simulink model "velo_pi_mbd_sl"  (R2023b)
settings: Solver=ode4  StartTime=0.0  StopTime=10  FixedStep=ts  RelTol=1e-3  EnableMultiTasking=on
values from neighbouring files (symbols this model uses):
  K = 0.625269    [model_data.mat]    (also in velo_id_verify.m)
  Ki = p1*p2*T/K    [velo_pi_mbd.m]
  Kp = - (T*(p1+p2)+1)/K    [velo_pi_mbd.m]
  T = 0.26    [model_data.mat]    (also in velo_id_verify.m)
  ts = 1/50    (= 0.02)    [velo_id_gain.m]    (also in velo_id_gain_cp.m; velo_id_tc.m; velo_pi_mbd.m)
  u_offset = 1.15936    [model_data.mat]    (also in velo_id_gain.m = -P(2) / P(1); velo_id_tc.m = (K_id*r_const - c1)/K_id; velo_id_verify.m)
libraries: arduinolib x2
settings Model: ExtModeTrigDuration=2  Creator=morita  LastModifiedBy=MunoLike
settings SolverCC: AlgebraicLoopSolver=TrustRegion
settings DataIOCC: SaveFormat=Array  ReturnWorkspaceOutputs=off
settings OptimizationCC: LifeSpan=1  MaxStackSize=64
settings DebuggingCC: UnconnectedInputMsg=warning  UnconnectedOutputMsg=warning  UnconnectedLineMsg=warning  SFUnexpectedBacktrackingDiag=warning  SFNoUnconditionalDefaultTransitionDiag=warning  ArithmeticOperatorsInVariantConditions=warning
settings HardwareCC: ProdBitPerInt=16  ProdBitPerPointer=16  ProdBitPerSizeT=16  ProdBitPerPtrDiffT=16  ProdLargestAtomicFloat=None  ProdWordSize=8  ProdHWDeviceType=Atmel->AVR  UseEmbeddedCoderFeatures=off  UseSimulinkCoderFeatures=off
settings ModelReferenceCC: EnableRefExpFcnMdlSchedulingChecks=on
settings SFSimCC: SimUseLocalCustomCode=off  CustomCodeUndefinedFunction=UseInterfaceOnly
settings RTWCC: Description=Embedded Coder  SystemTargetFile=ert.tlc  HardwareBoard=Arduino Uno  TemplateMakefile=ert_default_tmf  GenerateReport=on  RTWUseLocalCustomCode=off  Toolchain=Arduino AVR  BuildConfiguration=Faster Runs  LaunchReport=on
settings CodeAppCC: ForceParamTrailComments=on  OperatorAnnotations=on  StateflowObjectComments=on  MATLABSourceComments=on
settings ERTTargetCC: MultiwordLength=2048  ERTCustomFileBanners=off  SupportContinuousTime=on  SupportNonInlinedSFcns=on  SupportVariableSizeSignals=on  ModelStepFunctionPrototypeControlCompliant=off  ExtModeTransport=3  ExtModeStaticAlloc=on  ExtModeAutomaticAllocSize=off  ExtModeStaticAllocSize=250  ExtModeMexFile=ext_xcp  ExtModeIntrfLevel=Level2 - Open
settings ConfigComp: CovMetricSettings=dw  CovSaveCumulativeToWorkspaceVar=on  CovSaveSingleToWorkspaceVar=on  CovExternalEMLEnable=off

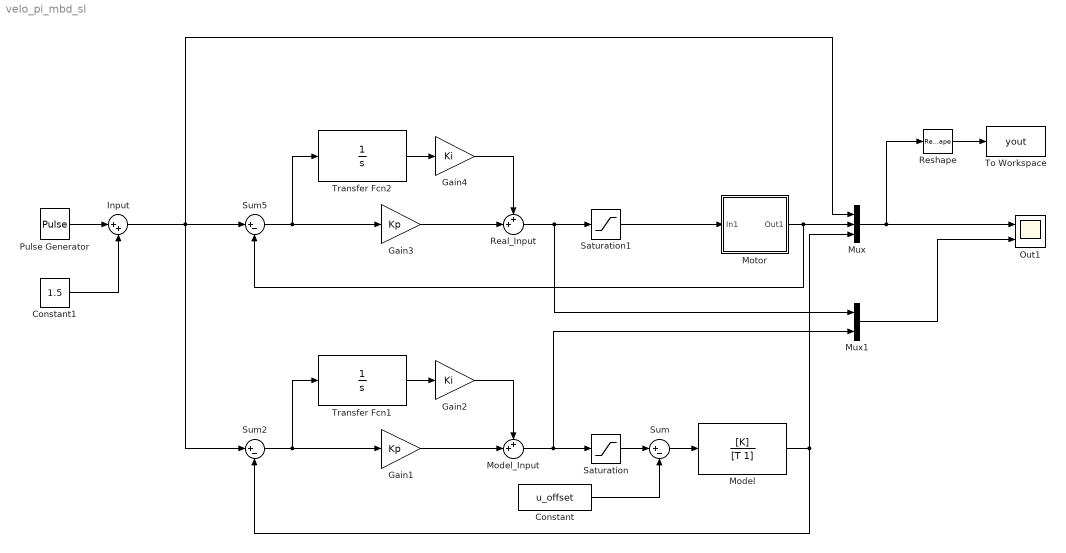
== system velo_pi_mbd_sl ==
  Constant : Constant  Value=u_offset
  Constant1 : Constant  Value=1.5
  Gain1 : Gain  Gain=Kp  ParamDataTypeStr=double  OutDataTypeStr=double
  Gain2 : Gain  Gain=Ki  ParamDataTypeStr=double  OutDataTypeStr=double
  Gain3 : Gain  Gain=Kp  ParamDataTypeStr=double  OutDataTypeStr=double
  Gain4 : Gain  Gain=Ki  ParamDataTypeStr=double  OutDataTypeStr=double
  Input : Sum  Inputs=|++
  Model : TransferFcn  Numerator=[K]  Denominator=[T 1]
  Model_Input : Sum  Inputs=++|
  Motor : Subsystem
  Mux : Mux  Inputs=3
  Mux1 : Mux  Inputs=2
  Out1 : Scope  NumInputPorts=2
  Pulse Generator : DiscretePulseGenerator  Amplitude=0.5  Period=4/ts  PulseWidth=2/ts  SampleTime=ts
  Real_Input : Sum  Inputs=++|
  Reshape : Reshape
  Saturation : Saturate  UpperLimit=5  LowerLimit=0
  Saturation1 : Saturate  UpperLimit=5  LowerLimit=0
  Sum : Sum  Inputs=|+-
  Sum2 : Sum  Inputs=|+-
  Sum5 : Sum  Inputs=|+-
  To Workspace : ToWorkspace  VariableName=yout  SaveFormat=Structure With Time  SampleTime=-1
  Transfer Fcn1 : TransferFcn  Denominator=[1 0]
  Transfer Fcn2 : TransferFcn  Denominator=[1 0]
  wires:
  Saturation1/1 -> Motor/1(In1)
  Reshape/1 -> To Workspace/1
  Constant/1 -> Sum/2
  Sum/1 -> Model/1
  Mux/1 -> Reshape/1, Out1/1
  Transfer Fcn1/1 -> Gain2/1
  Gain2/1 -> Model_Input/1
  Gain1/1 -> Model_Input/2
  Sum2/1 -> Transfer Fcn1/1, Gain1/1
  Model_Input/1 -> Mux1/2, Saturation/1
  Saturation/1 -> Sum/1
  Pulse Generator/1 -> Input/1
  Constant1/1 -> Input/2
  Model/1 -> Mux/3, Sum2/2
  Real_Input/1 -> Mux1/1, Saturation1/1
  Sum5/1 -> Gain3/1, Transfer Fcn2/1
  Gain3/1 -> Real_Input/2
  Gain4/1 -> Real_Input/1
  Transfer Fcn2/1 -> Gain4/1
  Motor/1(Out1) -> Mux/2, Sum5/2
  Input/1 -> Mux/1, Sum2/1, Sum5/1
  Mux1/1 -> Out1/2

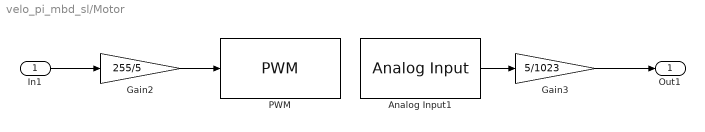
== system velo_pi_mbd_sl/Motor ==
  In1 : Inport
  Analog Input1 : arduinolib/Analog Input  pinNumber=0  ReadResultsOnly=off  ConversionTriggerSource=Software  ExternalTriggerType=uint32( 0 )  OutputDataType=uint16  EnableConversionCompleteNotify=off  EnableOuputStatus=off  SampleTime=ts  blockPlatform=arduino
  Gain2 : Gain  Gain=255/5  ParamDataTypeStr=double  OutDataTypeStr=double
  Gain3 : Gain  Gain=5/1023  ParamDataTypeStr=double  OutDataTypeStr=double
  PWM : arduinolib/PWM  pinNumber=3  frequencyType=Default  desiredFrequency=490.2  achievableFrequency=490.2
  Out1 : Outport  OutDataTypeStr=double
  wires:
  Analog Input1/1 -> Gain3/1
  Gain3/1 -> Out1/1
  Gain2/1 -> PWM/1
  In1/1 -> Gain2/1
